simulink library "adptfiltsubsys"  (Simulink 6.0)
values from neighbouring files (symbols this model uses):
  D = D + B    [rebuffer_delay.m]
  N = str2double(s)    [dspcsum.m]    (also in dspwdes.m = varargin{2}; if isempty(N), N=64; end; sdspmview2.m = size(cmap,1); sdspwfall.m = max(bd.indims))
undefined symbols (not defined in the file or in its folder): L, leakage
libraries: dspxfrm3 x5, dspsigops x4, dsparch4 x2, dspmtrx3 x2, dspindex x1, adptfiltsubsys x1
settings Model: Creator=navan  LastModifiedBy=sconahan

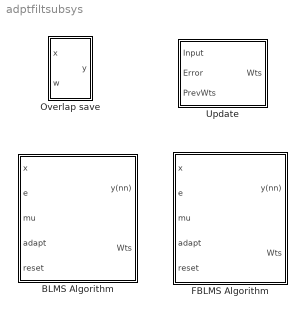
== system adptfiltsubsys ==
  BLMS Algorithm : Subsystem  mask(BLMS Algorithm){weights_algo=on}
      mask prompts: weights_algo "Output filter weights"
      mask help: Block LMS algorithm.
      mask init:
      | dspblkblmsalgo('blms');
  FBLMS Algorithm : Subsystem  mask(FBLMS Algorithm){weights_algo=on}
      mask prompts: weights_algo "Output filter weights"
      mask help: Fast Block LMS algorithm using FFT.
      mask init:
      | dspblkblmsalgo('fblms');
  Overlap save : Subsystem
  Update : Subsystem  mask(LMS based weight updates){Algo=LMS, stepflag=Dialog box, mu=0.1, leakage=1.0, Adapt=off, icw=0}
      mask prompts: Algo "Algorithm:"; stepflag "Specify step-size via:"; mu "Step-size, mu:"; leakage "Leakage factor (0 to 1):"; Adapt "Enable/disable adaptation via input port"; icw "Initial value of filter weights:"
      mask help: Weight update equlation for LMS based filters.
      mask init:
      | s=dspblklmsupdate('init');
      mask StyleString: popup(LMS|Normalized LMS|Sign-Error LMS|Sign-Data LMS|Sign-Sign LMS),popup(Dialog box|Input port),edit,edit,checkbox,edit
      mask CallbackString: |dspblklmsupdate('stepflag');|||dspblklmsupdate('init');|
      mask Display: disp(s);

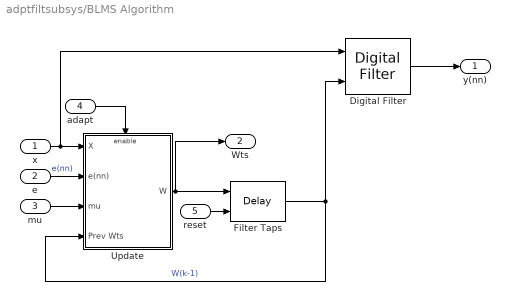
== system adptfiltsubsys/BLMS Algorithm ==
  x : Inport
  e : Inport  Port=2
  mu : Inport  Port=3
  adapt : Inport  Port=4
  reset : Inport  Port=5
  Digital Filter : dsparch4/Digital Filter  TypePopup=FIR (all zeros)  IIRFiltStruct=Direct form II transposed  AllPoleFiltStruct=Direct form  FIRFiltStruct=Direct form  CoeffSource=Input port(s)  NumCoeffs=[1 2]  DenCoeffs=[1 0.1]  BiQuadCoeffs=[1 0.3 0.4 1 0.1 0.2]  LatticeCoeffs=[0.2 0.4]  denIgnore=on  FiltPerSampPopup=One filter per frame  IC=0  ICnum=0  ICden=0  roundingMode=Floor  overflowMode=off
      settings: allowOverrides=off
  Filter Taps : dspsigops/Delay  dly_unit=Samples  delay=L  ic_detail=on  dif_ic_for_ch=off  dif_ic_for_dly=off  ic=ic  reset_popup=Non-zero sample
  Update : Subsystem
  y(nn) : Outport
  Wts : Outport  Port=2
  wires:
  Update/1(W) -> Filter Taps/1, Wts/1
  Filter Taps/1 -> Update/4(Prev Wts), Digital Filter/2  "W(k-1)"
  e/1 -> Update/2(e(nn))  "e(nn)"
  adapt/1 -> Update/Enable
  reset/1 -> Filter Taps/2
  x/1 -> Update/1(X), Digital Filter/1
  Digital Filter/1 -> y(nn)/1
  mu/1 -> Update/3(mu)

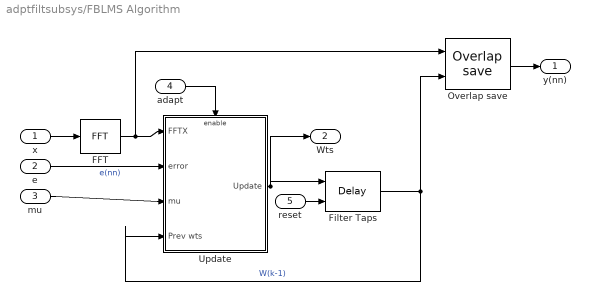
== system adptfiltsubsys/FBLMS Algorithm ==
  x : Inport
  e : Inport  Port=2
  mu : Inport  Port=3
  adapt : Inport  Port=4
  reset : Inport  Port=5
  FFT : dspxfrm3/FFT  CompMethod=Table lookup  TableOpt=Speed  BitRevOrder=off  SkipNorm=off  roundingMode=Floor  overflowMode=off
  Filter Taps : dspsigops/Delay  dly_unit=Samples  delay=L  ic_detail=on  dif_ic_for_ch=off  dif_ic_for_dly=off  ic=ic  reset_popup=Non-zero sample
  Overlap save : adptfiltsubsys/Overlap save
  Update : Subsystem
  y(nn) : Outport
  Wts : Outport  Port=2
  wires:
  reset/1 -> Filter Taps/2
  adapt/1 -> Update/Enable
  e/1 -> Update/2(error)  "e(nn)"
  Filter Taps/1 -> Overlap save/2, Update/4(Prev wts)  "W(k-1)"
  Update/1(Update) -> Filter Taps/1, Wts/1
  FFT/1 -> Update/1(FFTX), Overlap save/1
  x/1 -> FFT/1
  mu/1 -> Update/3(mu)
  Overlap save/1 -> y(nn)/1

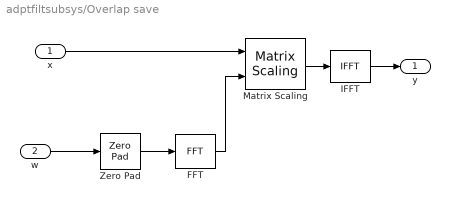
== system adptfiltsubsys/Overlap save ==
  x : Inport
  w : Inport  Port=2
  FFT : dspxfrm3/FFT  CompMethod=Table lookup  TableOpt=Speed  BitRevOrder=off  SkipNorm=off  roundingMode=Floor  overflowMode=off
  IFFT : dspxfrm3/IFFT  CompMethod=Table lookup  TableOpt=Speed  BitRevOrder=off  cs_in=off  SkipNorm=off  mode=Real  roundingMode=Floor  overflowMode=off
  Matrix Scaling : dspmtrx3/Matrix Scaling  mode=Scale rows (D*A)  D_Source=Input port  D_VectFromMask=[0.5 0.25]  roundingMode=Floor  overflowMode=off
  Zero Pad : dspsigops/Zero Pad  padSigAt=End  zpadAlong=Columns  padNumOutRowsSpecMethod=User-specified  numOutRows=L+N  padNumOutColsSpecMethod=User-specified  numOutCols=1  trunc_flag=None
  y : Outport
  wires:
  w/1 -> Zero Pad/1
  Zero Pad/1 -> FFT/1
  IFFT/1 -> y/1
  FFT/1 -> Matrix Scaling/2
  x/1 -> Matrix Scaling/1
  Matrix Scaling/1 -> IFFT/1

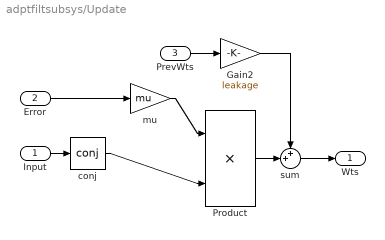
== system adptfiltsubsys/Update ==
  Input : Inport
  Error : Inport  Port=2
  PrevWts : Inport  Port=3
  Gain2 : Gain  Gain=leakage  SaturateOnIntegerOverflow=on
  Product : Product  SaturateOnIntegerOverflow=on
  conj : Math  Operator=conj  SaturateOnIntegerOverflow=on
  mu : Gain  Gain=mu  SaturateOnIntegerOverflow=on
  sum : Sum  Inputs=++|  SaturateOnIntegerOverflow=on  InputSameDT=on
  Wts : Outport  InitialOutput=icw(:)
  wires:
  mu/1 -> Product/1
  Error/1 -> mu/1
  conj/1 -> Product/2
  Input/1 -> conj/1
  sum/1 -> Wts/1
  Product/1 -> sum/2
  PrevWts/1 -> Gain2/1
  Gain2/1 -> sum/1

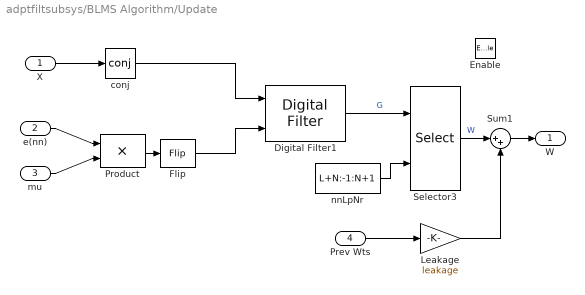
== system adptfiltsubsys/BLMS Algorithm/Update ==
  X : Inport
  e(nn) : Inport  Port=2
  mu : Inport  Port=3
  Prev Wts : Inport  Port=4
  Enable : EnablePort
  Digital Filter1 : dsparch4/Digital Filter  TypePopup=FIR (all zeros)  IIRFiltStruct=Direct form II transposed  AllPoleFiltStruct=Direct form  FIRFiltStruct=Direct form  CoeffSource=Input port(s)  NumCoeffs=[1 2]  DenCoeffs=[1 0.1]  BiQuadCoeffs=[1 0.3 0.4 1 0.1 0.2]  LatticeCoeffs=[0.2 0.4]  denIgnore=on  FiltPerSampPopup=One filter per frame  IC=0  ICnum=0  ICden=0  roundingMode=Floor  overflowMode=off
  Flip : dspindex/Flip  dim=Columns
  Leakage : Gain  Gain=leakage  SaturateOnIntegerOverflow=on
  Product : Product  SaturateOnIntegerOverflow=on  InputSameDT=on
  Selector3 : Selector  ElementSrc=External  Elements=[1 3]
  Sum1 : Sum  Inputs=|++  SaturateOnIntegerOverflow=on
  conj : Math  Operator=conj  SaturateOnIntegerOverflow=on
  nnLpNr : Constant  Value=L+N:-1:N+1
  W : Outport
  wires:
  Leakage/1 -> Sum1/2
  Sum1/1 -> W/1
  Selector3/1 -> Sum1/1  "W"
  Prev Wts/1 -> Leakage/1
  Digital Filter1/1 -> Selector3/1  "G"
  X/1 -> conj/1
  nnLpNr/1 -> Selector3/2
  conj/1 -> Digital Filter1/1
  Flip/1 -> Digital Filter1/2
  e(nn)/1 -> Product/1
  mu/1 -> Product/2
  Product/1 -> Flip/1

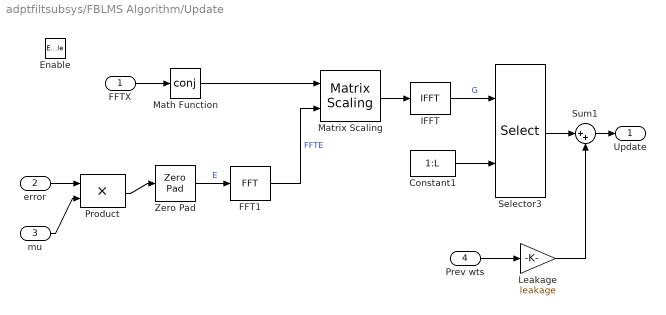
== system adptfiltsubsys/FBLMS Algorithm/Update ==
  FFTX : Inport
  error : Inport  Port=2
  mu : Inport  Port=3
  Prev wts : Inport  Port=4
  Enable : EnablePort
  Constant1 : Constant  Value=1:L
  FFT1 : dspxfrm3/FFT  CompMethod=Table lookup  TableOpt=Speed  BitRevOrder=off  SkipNorm=off  roundingMode=Floor  overflowMode=off
  IFFT : dspxfrm3/IFFT  CompMethod=Table lookup  TableOpt=Speed  BitRevOrder=off  cs_in=off  SkipNorm=off  mode=Real  roundingMode=Floor  overflowMode=off
  Leakage : Gain  Gain=leakage  SaturateOnIntegerOverflow=on
  Math Function : Math  Operator=conj  SaturateOnIntegerOverflow=on
  Matrix Scaling : dspmtrx3/Matrix Scaling  mode=Scale rows (D*A)  D_Source=Input port  D_VectFromMask=[0.5 0.25]  roundingMode=Floor  overflowMode=off
  Product : Product  SaturateOnIntegerOverflow=on  InputSameDT=on
  Selector3 : Selector  ElementSrc=External  Elements=[1 3]
  Sum1 : Sum  Inputs=|++  SaturateOnIntegerOverflow=on
  Zero Pad : dspsigops/Zero Pad  padSigAt=Beginning  zpadAlong=Columns  padNumOutRowsSpecMethod=User-specified  numOutRows=L+N  padNumOutColsSpecMethod=User-specified  numOutCols=1  trunc_flag=Error
  Update : Outport
  wires:
  FFTX/1 -> Math Function/1
  Constant1/1 -> Selector3/2
  Matrix Scaling/1 -> IFFT/1
  Math Function/1 -> Matrix Scaling/1
  FFT1/1 -> Matrix Scaling/2  "FFTE"
  Zero Pad/1 -> FFT1/1  "E"
  IFFT/1 -> Selector3/1  "G"
  Prev wts/1 -> Leakage/1
  Leakage/1 -> Sum1/2
  Selector3/1 -> Sum1/1
  Sum1/1 -> Update/1
  error/1 -> Product/1
  mu/1 -> Product/2
  Product/1 -> Zero Pad/1
